simulink model "SMO"  (R2020b)
settings: Solver=VariableStepAuto  StartTime=0.0  StopTime=10.0  RelTol=1e-3
undefined symbols (not defined in the file): l, Ls, Rs, SMO_h
libraries: dsparch4 x2, pid_lib x1
settings Model: Creator=Administrator  LastModifiedBy=Administrator

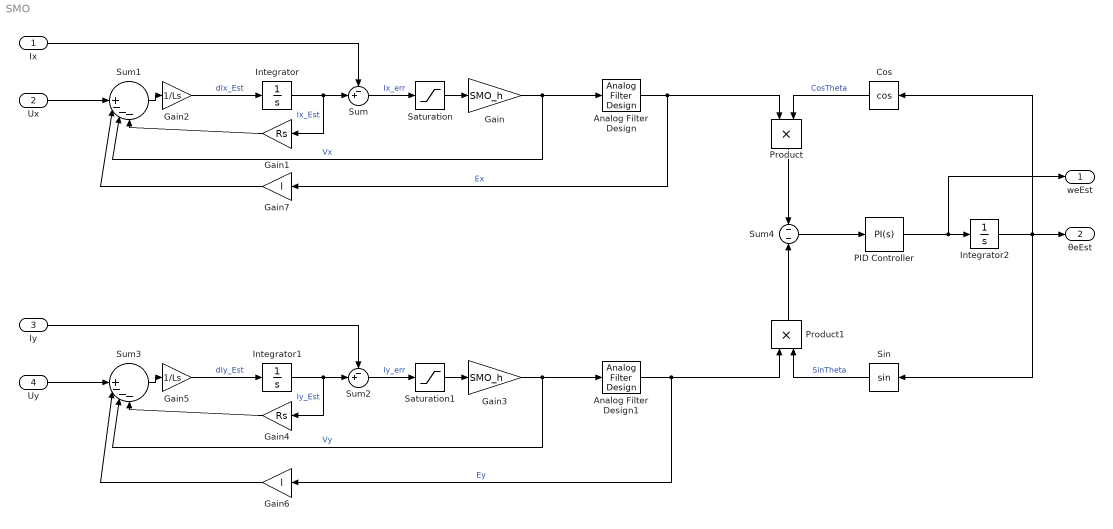
== system SMO ==
  Ix : Inport
  Ux : Inport  Port=2
  Iy : Inport  Port=3
  Uy : Inport  Port=4
  Analog Filter Design : dsparch4/Analog Filter Design  method=Butterworth  filttype=Lowpass  N=1  Wlo=2000*2*pi()  Whi=80  Rp=2  Rs=40
  Analog Filter Design1 : dsparch4/Analog Filter Design  method=Butterworth  filttype=Lowpass  N=1  Wlo=2000*2*pi()  Whi=80  Rp=2  Rs=40
  Cos : Trigonometry  Operator=cos
  Gain : Gain  Gain=SMO_h
  Gain1 : Gain  Gain=Rs
  Gain2 : Gain  Gain=1/Ls
  Gain3 : Gain  Gain=SMO_h
  Gain4 : Gain  Gain=Rs
  Gain5 : Gain  Gain=1/Ls
  Gain6 : Gain  Gain=l
  Gain7 : Gain  Gain=l
  Integrator : Integrator
  Integrator1 : Integrator
  Integrator2 : Integrator
  PID Controller : pid_lib/PID Controller  Controller=PI  Form=Parallel  TimeDomain=Continuous-time  UseExternalTs=off  SampleTime=-1  IntegratorMethod=Forward Euler  FilterMethod=Forward Euler  ControllerParametersSource=internal  P=1  I=1  D=0  UseFilter=on  N=100  TunerSelectOption=Transfer Function Based (PID Tuner App)  InitialConditionSource=internal  InitialConditionForIntegrator=0  InitialConditionForFilter=0  DifferentiatorICPrevScaledInput=0  ExternalReset=none  TrackingMode=off  Kt=1  LimitOutput=off  SatLimitsSource=internal  UpperSaturationLimit=inf  LowerSaturationLimit=-inf  LinearizeAsGain=on  AntiWindupMode=none  Kb=1  POutMin=[]  POutMax=[]  IOutMin=[]  IOutMax=[]  DOutMin=[]  DOutMax=[]  NOutMin=[]  NOutMax=[]  SumOutMin=[]  SumOutMax=[]  SaturationOutMin=[]  SaturationOutMax=[]  PParamMin=[]  PParamMax=[]  IParamMin=[]  IParamMax=[]  DParamMin=[]  DParamMax=[]  NParamMin=[]  NParamMax=[]  KbParamMin=[]  KbParamMax=[]  KtParamMin=[]  KtParamMax=[]  KbOutMin=[]  KbOutMax=[]  KtOutMin=[]  KtOutMax=[]  IntegratorOutMin=[]  IntegratorOutMax=[]  FilterOutMin=[]  FilterOutMax=[]  SumI1OutMin=[]  SumI1OutMax=[]  SumI2OutMin=[]  SumI2OutMax=[]  SumI3OutMin=[]  SumI3OutMax=[]  SumI4OutMin=[]  SumI4OutMax=[]  SumDOutMin=[]  SumDOutMax=[]  DifferentiatorOutMin=[]  DifferentiatorOutMax=[]  FilterDiffOutCoefMin=[]  FilterDiffOutCoefMax=[]  ReciprocalOutMin=[]  ReciprocalOutMax=[]  SumDenOutMin=[]  SumDenOutMax=[]  SumNumOutMin=[]  SumNumOutMax=[]  DivideOutMin=[]  DivideOutMax=[]  UdiffTsProdOutMin=[]  UdiffTsProdOutMax=[]  NTsProdOutMin=[]  NTsProdOutMax=[]  UintegralTsProdOutMin=[]  UintegralTsProdOutMax=[]  UngainTsProdOutMin=[]  UngainTsProdOutMax=[]  IntegratorContinuousStateAttributes=''  IntegratorStateMustResolveToSignalObject=off  IntegratorRTWStateStorageClass=Auto  FilterContinuousStateAttributes=''  FilterStateMustResolveToSignalObject=off  FilterRTWStateStorageClass=Auto  ParallelPVariant=InternalParameters  IdealPVariant=Disabled  IVariant=InternalParameters  DVariant=Disabled  IntegratorVariant=Continuous  SatVariant=Disabled  AWVariant=Passthrough  PCopyVariant=Disabled  TRVariant=Disabled  FdbkBlocksVariant=Forward  IdealPFdbkVariant=Disabled  SatFdbkVariant=Disabled  DerivativeFilterVariant=Disabled  NVariant=Disabled  NCopyVariant=Disabled_SignalSpec  FilterICVariant=Disabled  IntegratorICVariant=InternalICs  ExternalResetVariant=Disabled  TRSumVariant=Passthrough  SumFdbkVariant=Disabled  SumVariant=Sum_PI  TsampFilterVariant=InternalTs  TsampNgainVariant=Passthrough  TsampIntegralVariant=Passthrough  ExternalSaturationOutDataTypeStr=Inherit: Same as second input
  Product : Product
  Product1 : Product
  Saturation : Saturate
  Saturation1 : Saturate
  Sin : Trigonometry
  Sum : Sum  Inputs=-+|
  Sum1 : Sum  Inputs=|||+---
  Sum2 : Sum  Inputs=-+|
  Sum3 : Sum  Inputs=|||+---
  Sum4 : Sum  Inputs=-|-
  weEst : Outport
  θeEst : Outport  Port=2
  wires:
  Sum/1 -> Saturation/1  "Ix_err"
  Saturation/1 -> Gain/1
  Gain/1 -> Sum1/3, Analog Filter Design/1  "Vx"
  Integrator/1 -> Gain1/1, Sum/2  "Ix_Est"
  Sum1/1 -> Gain2/1
  Gain1/1 -> Sum1/4
  Gain2/1 -> Integrator/1  "dIx_Est"
  Analog Filter Design/1 -> Gain7/1, Product/1  "Ex"
  Ix/1 -> Sum/1
  Ux/1 -> Sum1/1
  Gain4/1 -> Sum3/4
  Sum3/1 -> Gain5/1
  Analog Filter Design1/1 -> Gain6/1, Product1/1  "Ey"
  Uy/1 -> Sum3/1
  Gain5/1 -> Integrator1/1  "dIy_Est"
  Iy/1 -> Sum2/1
  Sum2/1 -> Saturation1/1  "Iy_err"
  Integrator1/1 -> Gain4/1, Sum2/2  "Iy_Est"
  Gain3/1 -> Sum3/3, Analog Filter Design1/1  "Vy"
  Saturation1/1 -> Gain3/1
  Sin/1 -> Product1/2  "SinTheta"
  Cos/1 -> Product/2  "CosTheta"
  Product/1 -> Sum4/1
  Product1/1 -> Sum4/2
  Sum4/1 -> PID Controller/1
  PID Controller/1 -> weEst/1, Integrator2/1
  Integrator2/1 -> θeEst/1, Sin/1, Cos/1
  Gain6/1 -> Sum3/2
  Gain7/1 -> Sum1/2
